simulink model "test_multi_sample"  (Simulink 4.00)
settings: Solver=FixedStepDiscrete  StartTime=0.0  StopTime=10.0  FixedStep=0.01  RelTol=1e-3
settings Model: LastModifiedBy=bsaunder

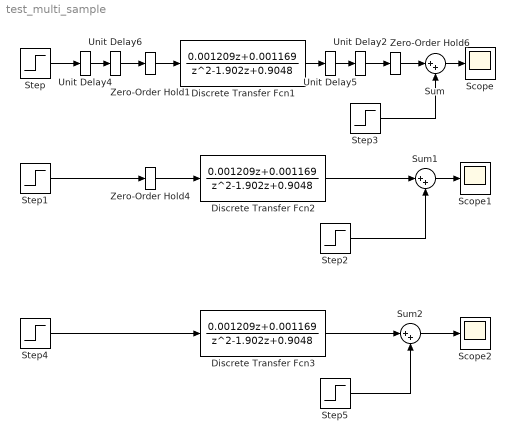
== system test_multi_sample ==
  Discrete Transfer Fcn1 : DiscreteTransferFcn  Numerator=[0.001209 0.001169]  Denominator=[1 -1.902 0.9048]  SampleTime=0.05  Realization=auto
      settings: RTWStateStorageClass=Auto
  Discrete Transfer Fcn2 : DiscreteTransferFcn  Numerator=[0.001209 0.001169]  Denominator=[1 -1.902 0.9048]  SampleTime=0.05  Realization=auto
      settings: RTWStateStorageClass=Auto
  Discrete Transfer Fcn3 : DiscreteTransferFcn  Numerator=[0.001209 0.001169]  Denominator=[1 -1.902 0.9048]  SampleTime=0.01  Realization=auto
      settings: RTWStateStorageClass=Auto
  Scope : Scope
      settings: TimeRange=10  YMin=0  YMax=1  SaveToWorkspace=off  SaveName=ScopeData  LimitDataPoints=on  MaxDataPoints=5000  SampleTime=0.02
  Scope1 : Scope
      settings: TimeRange=10  YMin=0  YMax=1  SaveToWorkspace=off  LimitDataPoints=on  MaxDataPoints=5000
  Scope2 : Scope
      settings: TimeRange=10  YMin=0  YMax=1  SaveToWorkspace=off  SaveName=ScopeData2  LimitDataPoints=on  MaxDataPoints=5000
  Step : Step  Time=2  Before=0  After=1  SampleTime=0.02
  Step1 : Step  Time=2  Before=0  After=1  SampleTime=0.01
  Step2 : Step  Time=8  Before=0  After=0  SampleTime=0.01
  Step3 : Step  Time=8  Before=0  After=0  SampleTime=0.02
  Step4 : Step  Time=2  Before=0  After=1  SampleTime=0.01
  Step5 : Step  Time=8  Before=0  After=0  SampleTime=0.01
  Sum : Sum  Inputs=|++  SaturateOnIntegerOverflow=on
  Sum1 : Sum  Inputs=|++  SaturateOnIntegerOverflow=on
  Sum2 : Sum  Inputs=|++  SaturateOnIntegerOverflow=on
  Unit Delay2 : UnitDelay  X0=0  SampleTime=0.01
      settings: RTWStateStorageClass=Auto
  Unit Delay4 : UnitDelay  X0=0  SampleTime=0.02
      settings: RTWStateStorageClass=Auto
  Unit Delay5 : UnitDelay  X0=0  SampleTime=0.05
      settings: RTWStateStorageClass=Auto
  Unit Delay6 : UnitDelay  X0=0  SampleTime=0.01
      settings: RTWStateStorageClass=Auto
  Zero-Order Hold1 : ZeroOrderHold  SampleTime=0.05
  Zero-Order Hold4 : ZeroOrderHold  SampleTime=0.05
  Zero-Order Hold6 : ZeroOrderHold  SampleTime=0.02
  wires:
  Step/1 -> Unit Delay4/1
  Discrete Transfer Fcn1/1 -> Unit Delay5/1
  Unit Delay5/1 -> Unit Delay2/1
  Zero-Order Hold1/1 -> Discrete Transfer Fcn1/1
  Unit Delay4/1 -> Unit Delay6/1
  Unit Delay6/1 -> Zero-Order Hold1/1
  Step1/1 -> Zero-Order Hold4/1
  Zero-Order Hold4/1 -> Discrete Transfer Fcn2/1
  Sum/1 -> Scope/1
  Zero-Order Hold6/1 -> Sum/1
  Sum1/1 -> Scope1/1
  Discrete Transfer Fcn2/1 -> Sum1/1
  Step2/1 -> Sum1/2
  Step3/1 -> Sum/2
  Step4/1 -> Discrete Transfer Fcn3/1
  Sum2/1 -> Scope2/1
  Discrete Transfer Fcn3/1 -> Sum2/1
  Step5/1 -> Sum2/2
  Unit Delay2/1 -> Zero-Order Hold6/1
